simulink model "ModelBlocks"  (R2023a)
settings: Solver=daessc  StartTime=0.0  StopTime=6  FixedStep=1e-4  RelTol=1e-4
model workspace (MAT data in the model file):
  N_p0 = 5
  N_v0 = 0
  N_w0 = 0
  t_ion = 0
  t_p = 12
  t_pump = 32
  t_release = 5
  t_retention = 2
undefined symbols (not defined in the file): Nv0, par0
settings Model: ParameterArgumentNames=N_p0,N_v0,N_w0,t_ion,t_p,t_pump,t_release,t_retention  Creator=levsi  LastModifiedBy=levsi
settings SolverCC: MaxConsecutiveMinStep=10  ODENIntegrationMethod=ode14x
settings DataIOCC: ReturnWorkspaceOutputs=off

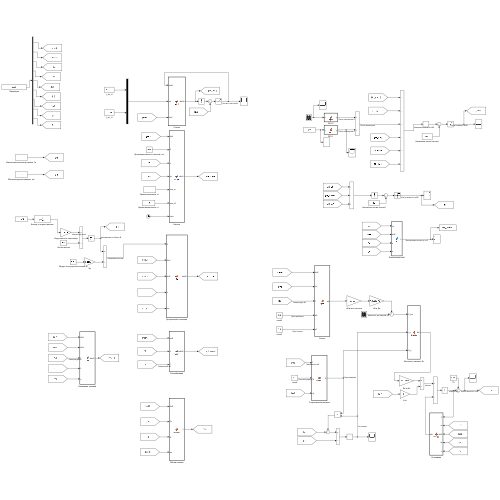
[thumbnail: Simulink's stored preview of the top-level diagram]
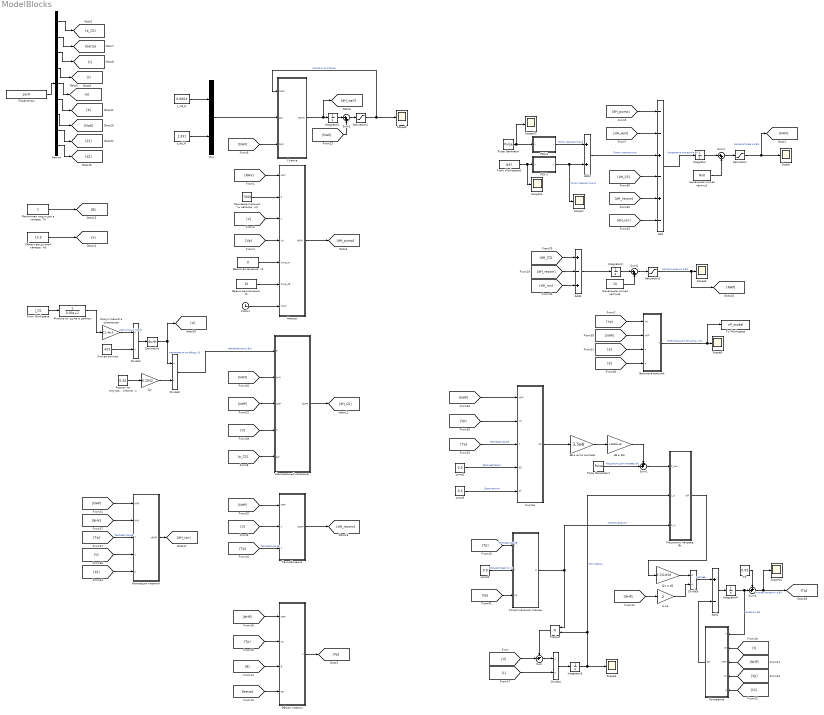
== system ModelBlocks ==
  2pi : Gain  Gain=6.2832
  Add : Sum  Inputs=--+-+-
  Add1 : Sum  Inputs=+-
  Add2 : Sum
  Add3 : Sum  Inputs=+-+
  Clock1 : Clock
  Demux : Demux  Outputs=9
  Derivative : Derivative
  Divide{2..5} (4 alike) : Product  Inputs=*/
  From Workspace : FromWorkspace  VariableName=I_CS  OutputAfterFinalValue=Holding final value
  From Workspace2 : FromWorkspace  VariableName=gas  OutputAfterFinalValue=Holding final value
  H+e : Gain  Gain=2
  Integrator{,1..2,4} (4 alike) : Integrator  LowerSaturationLimit=0
  Integrator3 : Integrator
  Mux : Mux  Inputs=2
  PEV-1 : MATLAB Function  TreatAsAtomicUnit=on
  PEV-3 : MATLAB Function  TreatAsAtomicUnit=on
  Product : Product
  Pulse Generator : DiscretePulseGenerator  PulseType=Time based  Amplitude=35.8  Period=1  PulseWidth=50
  Pulse Generator1 : DiscretePulseGenerator  PulseType=Time based  Amplitude=0  Period=100  PhaseDelay=2
  Saturation : Saturate  UpperLimit=1e30  LowerLimit=0
  Saturation1 : Saturate  UpperLimit=1e30  LowerLimit=0
  Saturation2 : Saturate  UpperLimit=1e30  LowerLimit=0
  Scope{,1..3,6..7,10..11,16} (9 alike) : Scope
  Sum : Sum  Inputs=-+|
  Sum1 : Sum  Inputs=++|
  Sum2 : Sum  Inputs=|++
  Sum3 : Sum  Inputs=|++
  Sum4 : Sum  Inputs=++|
  Sum6 : Sum  Inputs=|++
  T0 : Constant  Value=0.03
  To Workspace : ToWorkspace  VariableName=nP_model  SaveFormat=Timeseries  SampleTime=0.001
  const2 : Constant  Value=0.5
  const3 : Constant  Value=0.5
  const4 : Constant  Value=0.9
  t_rel_H : Constant  Value=1.331
  t_ret_H : Constant  Value=0.0003
  "Время включения, с1" : Constant  Value=0
  "Время выключения, с1" : Constant  Value=10
  Вспомогательный : MATLAB Function  TreatAsAtomicUnit=on
  Дж в эВ : Gain  Gain=6.2414e18
  Индуктивность соленоида : Gain  Gain=11.4e-3
  Ионизация плазмой : MATLAB Function  TreatAsAtomicUnit=on
  Кол-во витков : Constant  Value=423
  "Магнитная индукция в камере, Тл" : Constant
  "Мощность нагрева, Вт" : MATLAB Function  TreatAsAtomicUnit=on
  Насосы : MATLAB Function  TreatAsAtomicUnit=on
  Начальное кол-во частиц1 : Constant  Value=Nv0
  Начальное кол-во частиц3 : Constant  Value=10
  "Объем вакуумной камеры, м3 " : Constant  Value=13.5
  Объем плазмы : MATLAB Function  TreatAsAtomicUnit=on
  Остывание : MATLAB Function  TreatAsAtomicUnit=on
  Параметры : Constant  Value=par0
  "Производительность насосов, л/с" : Constant  Value=7600
  "Радиус по внутренней стенке, м" : Constant  Value=0.45
  Рекомбинация : MATLAB Function  TreatAsAtomicUnit=on
  Синтез : MATLAB Function  TreatAsAtomicUnit=on
  Сопротивление пламзы : MATLAB Function  TreatAsAtomicUnit=on
  Стенка : MATLAB Function  TreatAsAtomicUnit=on
  Фильтр от шума в данных : TransferFcn  Denominator=[0.03 1]
  Центральный соленоид : MATLAB Function  TreatAsAtomicUnit=on
  эВ в Дж : Gain  Gain=1.6022e-19
  эВ в акте синтеза : Gain  Gain=3.5e6
  wires:
  Integrator/1 -> Sum2/1
  Sum2/1 -> Saturation/1
  Saturation/1 -> [NHV], Scope/1  "Кол-во атомов H в ВК"
  Saturation1/1 -> Стенка/1(NHW), Scope2/1  "Кол-во H на стенке"
  Integrator1/1 -> Sum3/1
  Sum3/1 -> Saturation1/1
  Add/1 -> Integrator/1  "Изменение кол-ва H в ВК"
  Add3/1 -> Integrator2/1
  "Магнитная индукция в камере, Тл"/1 -> [B]
  "Объем вакуумной камеры, м3 "/1 -> [V]
  Clock1/1 -> Насосы/7(clock)
  "Время выключения, с1"/1 -> Насосы/6(time_off)
  "Время включения, с1"/1 -> Насосы/5(time_on)
  "Производительность насосов, л/с"/1 -> Насосы/2(S)
  Вспомогательный/1(Y) -> To Workspace/1, Scope6/1  "Электронная плотность, м-3"
  Saturation2/1 -> Scope1/1, [NHP]  "Кол-во ионов H+ в ВК"
  Mux/1 -> Стенка/2(par)
  t_ret_H/1 -> Mux/1
  t_rel_H/1 -> Mux/2
  PEV-3/1(y) -> Add2/1  "Поток газонапуска H"
  PEV-1/1(y) -> Scope7/1, Add2/2  "Поток газонапуска H"
  Pulse Generator/1 -> Scope10/1, PEV-3/1(u)
  From Workspace2/1 -> Scope11/1, PEV-1/1(u)
  Integrator2/1 -> Sum6/1
  Sum6/1 -> Saturation2/1
  Начальное кол-во частиц3/1 -> Sum6/2
  [V] -> Насосы/3(V)
  [Vp] -> Насосы/4(Vp)
  Насосы/1(dNHV) -> [dH_pump]
  [NHV] -> Насосы/1(NHV)
  [NHV] -> Стенка/3(NHV)
  Стенка/1(dNHW) -> [dH_wall], Integrator1/1
  Derivative/1 -> Divide3/1, [U]  "Напряжение по обходу, В"
  Divide2/1 -> Derivative/1
  Индуктивность соленоида/1 -> Divide2/1  "Магнитный поток"
  Кол-во витков/1 -> Divide2/2
  2pi/1 -> Divide3/2
  "Радиус по внутренней стенке, м"/1 -> 2pi/1
  Divide3/1 -> Центральный соленоид/1(E)  "Напряженность В/м"
  [V] -> Центральный соленоид/4(V)
  [NHP] -> Центральный соленоид/3(NHP)
  [NHV] -> Центральный соленоид/2(NHV)
  Центральный соленоид/1(dNHP) -> [dH_CS]
  Фильтр от шума в данных/1 -> Индуктивность соленоида/1
  From Workspace/1 -> Фильтр от шума в данных/1
  Рекомбинация/1(dNHP) -> [dH_recom]
  [NHP] -> Рекомбинация/1(NHP)
  [NHP] -> Синтез/1(NHP)
  [Vp] -> Синтез/2(Vp)
  const2/1 -> Синтез/4(dD)  "Доля дейтерия"
  const3/1 -> Синтез/5(dT)  "Доля трития"
  Синтез/1(dN) -> эВ в акте синтеза/1
  [Tp] -> Сопротивление пламзы/1(T)  "Температура эВ"
  const4/1 -> Сопротивление пламзы/2(r)  "Большой радиус, м"
  [Vp] -> Сопротивление пламзы/3(Vp)
  эВ в акте синтеза/1 -> эВ в Дж/1
  эВ в Дж/1 -> Sum1/1
  Сопротивление пламзы/1(R) -> "Мощность нагрева, Вт"/3(R_p), Product/1  "Сопротивление"
  Pulse Generator1/1 -> Sum1/2  "Мощность доп нагрева, Вт"
  Sum1/1 -> "Мощность нагрева, Вт"/1(P_aux)
  [B] -> Объем плазмы/3(B)
  [betta] -> Объем плазмы/4(par)
  [Tp] -> Объем плазмы/2(Tp)
  [NHP] -> Объем плазмы/1(NHP)
  Объем плазмы/1(V) -> [Vp]
  [Vp] -> Вспомогательный/1(Vp)
  [NHP] -> Вспомогательный/2(NHP)
  [Tp] -> Рекомбинация/3(T)  "Температура эВ"
  H+e/1 -> Divide5/2
  [NHP] -> H+e/1
  Дж в эВ/1 -> Divide5/1
  "Мощность нагрева, Вт"/1(dW) -> Дж в эВ/1
  Divide5/1 -> Add1/1  "Нагрев"
  Add1/1 -> Integrator4/1
  Integrator4/1 -> Остывание/1(T), Sum4/2  "Энергия. эВ"
  [V] -> Рекомбинация/2(V)
  Параметры/1 -> Demux/1
  [a_CS] -> Центральный соленоид/5(par)
  [Nw0] -> Sum3/2
  Начальное кол-во частиц1/1 -> Sum2/2
  [dH_wall] -> Add/2
  Add2/1 -> Add/3  "Поток газонапуска"
  [dH_pump] -> Add/1
  [dH_CS] -> Add3/1
  Demux/4 -> [t]
  Demux/3 -> [L]
  Demux/2 -> [betta]
  Demux/1 -> [a_CS]
  [U] -> Sum/2
  Product/1 -> Sum/1
  Sum/1 -> Divide4/1
  [L] -> Divide4/2
  Divide4/1 -> Integrator3/1
  Integrator3/1 -> Scope3/1, "Мощность нагрева, Вт"/2(I_p), Product/2  "Ток плазмы"
  Sum4/1 -> Scope16/1, [Tp]  "Кол-во ионов H+ в ВК"
  T0/1 -> Sum4/1
  [t] -> Остывание/2(te)
  Остывание/1(dW) -> Add1/2
  [NHP] -> Остывание/3(NHP)
  [Vp] -> Остывание/4(Vp)
  [dH_CS] -> Add/4
  [Tp] -> Синтез/3(T)  "Температура эВ"
  [k1] -> Остывание/5(a)
  [Tp] -> Ионизация плазмой/3(T)  "Температура эВ"
  [NHP] -> Ионизация плазмой/1(NHP)
  [V] -> Ионизация плазмой/4(V)
  [NHV] -> Ионизация плазмой/2(NHV)
  [k2] -> Ионизация плазмой/5(q)
  Ионизация плазмой/1(dNHP) -> [dH_ion]
  Demux/7 -> [Nw0]
  Demux/5 -> [a]
  Demux/6 -> [b]
  [a] -> Вспомогательный/3(a)
  [b] -> Вспомогательный/4(b)
  [dH_recom] -> Add3/2
  [dH_recom] -> Add/5
  Demux/8 -> [k1]
  Demux/9 -> [k2]
  [dH_ion] -> Add3/3
  [dH_ion] -> Add/6

== matlab function ModelBlocks/Стенка ==
  data: dNHW output; NHW input; par input; NHV input
function dNHW= wall(NHW, par, NHV)

%% Константы
t_retention_H = par(1); %постоянная времени поглощения H
t_release_H = par(2); %постоянная времени выхода H

%%
dNHW = NHV / t_retention_H - NHW / t_release_H;

end

== matlab function ModelBlocks/Рекомбинация ==
  data: dNHP output; NHP input; V input; T input
function dNHP = recom(NHP, V, T)

%Расчет рекомбинации
y_vals = [7e-13 3.3249e-13 2.4658e-13 1.1675e-13 4.9391e-14 1.3333e-14 2.8735e-15 5.7433e-16 1.5764e-17 4.0135e-19 1.4e-20 1e-22 1e-40];
x_vals = [0.01 1.0328 1.5891 4.2339 11.287 44.5668 176.197 644.57 8988.46 1.206e5 1.206e6 1.2e8 1e20];
q = interp1(x_vals, y_vals, T); %скорость рекомбинации см3с-1
q = q*1e6; %скорость рекомбинации м3с-1

dNHP = q * (NHP/V) * NHP; %рекомбинация

end

== matlab function ModelBlocks/Центральный соленоид ==
  data: E input; NHV input; NHP input; V input; par input; dNHP output
function dNHP = CS(E, NHV, NHP, V, par)

    %Константы и параметры
    a_CS = par(1);
    e = 1.6022e-19; %заряд электрона, Кл
    m = 9.1094e-31; %масса электрона, кг
  
    %Расчет
    E = abs(E);
    n = (NHV + NHP) / V; %концентрация ядер м-3
    l = a_CS / n; %длина свободного пробега электрона, м
    W1 = E * l; %энергия, которую преобрел электрон за длину свободного пробега, эВ
    W2 = e * E * l; %энергия, которую преобрел электрон за длину свободного пробега, Дж
    
    if W1>0
        q = (1e-19)*((2.9e3)/(W1) * exp(-15/sqrt(W1))); %сечение ионизации, м2
        nH = NHV/V; %концентрация H, м-3
        ne = NHP/V; %концентрация e, м-3
        ve = sqrt(2 * W2 / m);% скорость е, м/с
    else
        q = 0;
        nH = 0;
        ne = 0;
        ve = 0;
    end

    dNHP = nH * ne * ve * q * V;

end

== matlab function ModelBlocks/Синтез ==
  data: dN output; NHP input; Vp input; T input; dD input; dT input
function dN  = synt(NHP, Vp, T, dD, dT)

%Константы
mD = 3.3436e-27; %масса дейтрона, кг
mT = 5.0072e-27; %масса тритона, кг
e = 1.6022e-19; %заряд электрона, Кл

%Расчет
vD =  sqrt(2 * (T * e) / mD); %скорость ядер Дейтерия, м/с
vT =  sqrt(2 * (T * e) /  mT); %скорость ядер Трития, м/с
v = (vD + vT) / 2; %средняя скорость ядер
T = T/1000; %Температура плазмы, кэВ
q = 2e-4/T * exp(-46/sqrt(T)); %сечение реакции DT, барн
q = q * 1e-28; %сечение реакции DT, м2

dN = q * (dD*NHP) * (dT*NHP) * v / Vp; %скорость реакции в объеме плазмы

end

== matlab function ModelBlocks/Сопротивление пламзы ==
  data: T input; r input; Vp input; R output
function R = current(T, r, Vp)

%Расчет
T = T / 1000; %температура кэВ
p = 2.4e-2/(T^(3/2)); %удельное сопротивление плазмы, мкОм мм2 м-1
p = p * 1e-6 / (1000 * 1000); %удельное сопротивление плазмы, Ом м2 м-1

l = 2 * pi * r; %длина окружности по большому радиусу, м
R = p * l * l / Vp; %сопротивление плазменного шнура, Ом

end

== matlab function ModelBlocks/Мощность нагрева, Вт ==
  data: dW output; P_aux input; I_p input; R_p input
function dW  = energy(P_aux, I_p, R_p)

%Расчет
P_current = R_p * I_p^2; %мощность омического нагрева, Вт
dW = P_current + P_aux;

end

== matlab function ModelBlocks/Вспомогательный ==
  data: Y output; Vp input; NHP input; a input; b input
function Y  = A(Vp, NHP, a, b)

q = 1 / (1 + exp(a * b - b * NHP)); %чувствительность прибора

Y = q * NHP / Vp;

end

== matlab function ModelBlocks/Остывание ==
  data: dW output; T input; te input; NHP input; Vp input; a input
function dW  = energy(T, te, NHP, Vp, a)

%Расчет
Pe = T / te; %энергетическое время жизни
Prad = a * NHP * T / Vp; %радиационные потери
dW = Pe + Prad;

end

== matlab function ModelBlocks/Ионизация плазмой ==
  data: dNHP output; NHP input; NHV input; T input; V input; q input
function dNHP = ion(NHP, NHV, T, V, q)

%Расчет ионизации
y_vals = [0.01e-18 0.2e-18 0.4e-18 1e-18 2e-18 5e-18 12e-18 20e-18 30e-18];
x_vals = [0 1000 2000 3000 4000 5000 8000 11000 14000];
Q = interp1(x_vals, y_vals, T);%см2
Q = Q / 1e4;%м2

dNHP = q * Q * (NHV/V) * NHP * sqrt(T);

end

== matlab function ModelBlocks/Объем плазмы ==
  data: V output; NHP input; Tp input; B input; par input
function V  = volume(NHP, Tp, B, par)

%Параметры и константы
b = par(1); %параметр бетта
k = 1.3806e-23; %постоянная Больцмана

%Расчет
N = NHP; %Кол-во ядер в плазме
T = Tp * 11640; %температура плазмы, К;
P = 0.4 * B^2 * 1e6; %давление магнитного поля, Па
V = N * k * T / b / P;

end

== matlab function ModelBlocks/Насосы ==
  data: NHV input; S input; dNHV output; V input; Vp input; time_on input; time_off input; clock input
function dNHV = pump(NHV, S, V, Vp, time_on, time_off, clock)

t_pump = (V-Vp) * 1000 / S;

if clock > time_on && clock < time_off
    dNHV = NHV / t_pump;
else
    dNHV = 0;
end

end

== matlab function ModelBlocks/PEV-1 ==
  data: u input; y output
function y = PEV(u)
    y_vals = [0, 18, 28, 42, 62, 80, 100, 123, 154, 180, 200, 232, 259, 280, 300, 323, 346, 360, 400, 433, 450, 478, 500, 538, 552, 580, 600, 635, 668, 700, 729, 750, 770, 800, 839, 870, 900, 930, 958, 988, 1000, 1050, 1100];
    x_vals = [20, 32, 35, 40, 44.8, 48.2, 50, 52.2, 54.8, 56.5, 57.5, 60, 61.7, 62.8, 63.9, 65, 66.1, 67.5, 70, 71, 72, 74, 75, 76.5, 78, 80, 82, 83, 85, 87, 88, 90, 90.8, 91.8, 93, 94.5, 96.2, 97.2, 98, 98.2, 98.5, 98.8, 99];
    if (u >= x_vals(1))
        Gase = interp1(x_vals, y_vals, u);
    else
        Gase = 0;
    end
    y = 2 * Gase * 0.0980665*6.02e23/(60*8.31*300);
end

== matlab function ModelBlocks/PEV-3 ==
  data: u input; y output
function y = PEV(u)
    y_vals = [0, 18, 28, 42, 62, 80, 100, 123, 154, 180, 200, 232, 259, 280, 300, 323, 346, 360, 400, 433, 450, 478, 500, 538, 552, 580, 600, 635, 668, 700, 729, 750, 770, 800, 839, 870, 900, 930, 958, 988, 1000, 1050, 1100];
    x_vals = [20, 32, 35, 40, 44.8, 48.2, 50, 52.2, 54.8, 56.5, 57.5, 60, 61.7, 62.8, 63.9, 65, 66.1, 67.5, 70, 71, 72, 74, 75, 76.5, 78, 80, 82, 83, 85, 87, 88, 90, 90.8, 91.8, 93, 94.5, 96.2, 97.2, 98, 98.2, 98.5, 98.8, 99];
    if (u >= x_vals(1))
        Gase = interp1(x_vals, y_vals, u);
    else
        Gase = 0;
    end
    y = 2 * Gase * 0.0980665*6.02e23/(60*8.31*300);
end
